simulink model "ayaz_th"  (R2018b)
settings: Solver=ode15s  StartTime=0.0  StopTime=duration_s  MaxStep=5  RelTol=1e-3  AbsTol=1e-3
undefined symbols (not defined in the file or in its folder): unstretched_l
libraries: origionalPlant x1, ayazController_cl x1, ayazWinches_cl x1
settings Model: Creator=mcobb  LastModifiedBy=mcobb

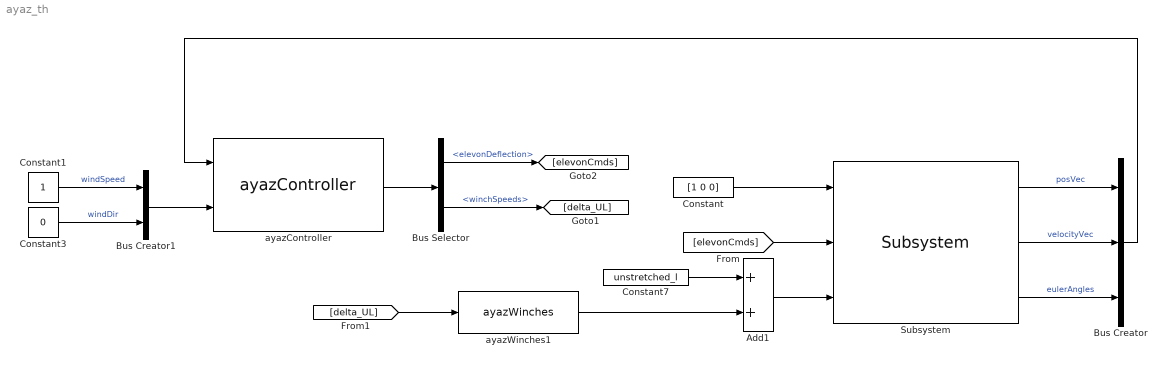
== system ayaz_th ==
  Add1 : Sum
  Bus Creator : BusCreator  Inputs=3  OutDataTypeStr=Bus: plantBus
  Bus Creator1 : BusCreator  Inputs=2  OutDataTypeStr=Bus: envBus
  Bus Selector : BusSelector  OutputSignals=elevonDeflection,winchSpeeds
  Constant : Constant  Value=[1 0 0]
  Constant1 : Constant
  Constant3 : Constant  Value=0
  Constant7 : Constant  Value=unstretched_l
  Subsystem : origionalPlant/Subsystem  SystemSampleTime=-1
  ayazController : ayazController_cl/ayazController  SystemSampleTime=-1  VariantControl=VSS_controller_ayazController
  ayazWinches1 : ayazWinches_cl/ayazWinches  SystemSampleTime=-1
  wires:
  Constant/1 -> Subsystem/1
  [elevonCmds] -> Subsystem/2
  Constant7/1 -> Add1/1
  ayazWinches1/1 -> Add1/2
  Add1/1 -> Subsystem/3
  ayazController/1 -> Bus Selector/1
  Bus Selector/2 -> [delta_UL]  "<winchSpeeds>"
  Bus Selector/1 -> [elevonCmds]  "<elevonDeflection>"
  [delta_UL] -> ayazWinches1/1
  Bus Creator/1 -> ayazController/1
  Bus Creator1/1 -> ayazController/2
  Constant1/1 -> Bus Creator1/1  "windSpeed"
  Constant3/1 -> Bus Creator1/2  "windDir"
  Subsystem/1 -> Bus Creator/1  "posVec"
  Subsystem/2 -> Bus Creator/2  "velocityVec"
  Subsystem/3 -> Bus Creator/3  "eulerAngles"
